simulink library "gmp_std_model_pck"  (R2024b)
settings: Solver=VariableStepAuto  StartTime=0.0  StopTime=10.0  RelTol=1e-3
undefined symbols (not defined in the file or in its folder): gcbh, sps_rtmsupport
libraries: spsSeriesRLCBranchLib x45, gmp_peripheral_utilities x32, spsVoltageMeasurementLib x21, spsSecondOrderFilterLib x19, spsMosfetLib x8, spsCurrentMeasurementLib x4, peripheral_utilities x3, gmp_fp_utilities x2, simulink x2
(part 3 of 5)

== system gmp_std_model_pck/Three Phase Bridge Ideal Current Measurement ==
  note: →
  note: Javnson
      | 2024.08.29
  note: GMP (General Motor Platform)
      | Simulink Toolkits
  note: current positive direction
  Trigger : Inport
  Ideal Current Measurement Module（ADC - Current）-U : gmp_peripheral_utilities/Ideal Current Measurement Module (ADC - Current)  ADC_GAIN=ADC_GAIN  ADC_BIT=ADC_BIT  ADC_REFERENCE=ADC_REFERENCE  ADC_BIAS=ADC_BIAS  ADC_INIT=ADC_INIT
      settings: SourceProductName=Virtual Peripheral Utilities
  Ideal Current Measurement Module（ADC - Current）-V : gmp_peripheral_utilities/Ideal Current Measurement Module (ADC - Current)  ADC_GAIN=ADC_GAIN  ADC_BIT=ADC_BIT  ADC_REFERENCE=ADC_REFERENCE  ADC_BIAS=ADC_BIAS  ADC_INIT=ADC_INIT
      settings: SourceProductName=Virtual Peripheral Utilities
  Ideal Current Measurement Module（ADC - Current）-W : gmp_peripheral_utilities/Ideal Current Measurement Module (ADC - Current)  ADC_GAIN=ADC_GAIN  ADC_BIT=ADC_BIT  ADC_REFERENCE=ADC_REFERENCE  ADC_BIAS=ADC_BIAS  ADC_INIT=ADC_INIT
      settings: SourceProductName=Virtual Peripheral Utilities
  Mux3 : Mux  Inputs=3
  Mux4 : Mux  Inputs=3
  Mux5 : Mux  Inputs=3
  A+ : PMIOPort  Side=Left
  B+ : PMIOPort  Port=2  Side=Left
  C+ : PMIOPort  Port=3  Side=Left
  a- : PMIOPort  Port=4  Side=Right
  b- : PMIOPort  Port=5  Side=Right
  c- : PMIOPort  Port=6  Side=Right
  Current ADC Sample Result : Outport
  Current ADC Scope(p.u.) : Outport  Port=2
  Current Real Value & HS : Outport  Port=3
  wires:
  [PhaseA_current] -> Mux3/1
  [PhaseB_current] -> Mux3/2
  [PhaseC_current] -> Mux3/3
  Mux3/1 -> Current ADC Sample Result/1
  [Ph_A_pu] -> Mux4/1
  [Ph_B_pu] -> Mux4/2
  [Ph_C_pu] -> Mux4/3
  Mux4/1 -> Current ADC Scope(p.u.)/1
  [Ph_B_HS] -> Mux5/2
  Mux5/1 -> Current Real Value & HS/1
  [Ph_C_HS] -> Mux5/3
  [Ph_A_HS] -> Mux5/1
  Trigger/1 -> Ideal Current Measurement Module（ADC - Current）-W/1, Ideal Current Measurement Module（ADC - Current）-V/1, Ideal Current Measurement Module（ADC - Current）-U/1
  Ideal Current Measurement Module（ADC - Current）-U/1 -> [PhaseA_current]
  Ideal Current Measurement Module（ADC - Current）-U/2 -> [Ph_A_pu]
  Ideal Current Measurement Module（ADC - Current）-U/3 -> [Ph_A_HS]
  Ideal Current Measurement Module（ADC - Current）-V/1 -> [PhaseB_current]
  Ideal Current Measurement Module（ADC - Current）-V/2 -> [Ph_B_pu]
  Ideal Current Measurement Module（ADC - Current）-V/3 -> [Ph_B_HS]
  Ideal Current Measurement Module（ADC - Current）-W/1 -> [PhaseC_current]
  Ideal Current Measurement Module（ADC - Current）-W/2 -> [Ph_C_pu]
  Ideal Current Measurement Module（ADC - Current）-W/3 -> [Ph_C_HS]
  connections:
  Ideal Current Measurement Module（ADC - Current）-U/LConn1 -- A+/RConn1
  Ideal Current Measurement Module（ADC - Current）-U/RConn1 -- a-/RConn1
  Ideal Current Measurement Module（ADC - Current）-V/RConn1 -- b-/RConn1
  Ideal Current Measurement Module（ADC - Current）-V/LConn1 -- B+/RConn1
  Ideal Current Measurement Module（ADC - Current）-W/RConn1 -- c-/RConn1
  Ideal Current Measurement Module（ADC - Current）-W/LConn1 -- C+/RConn1

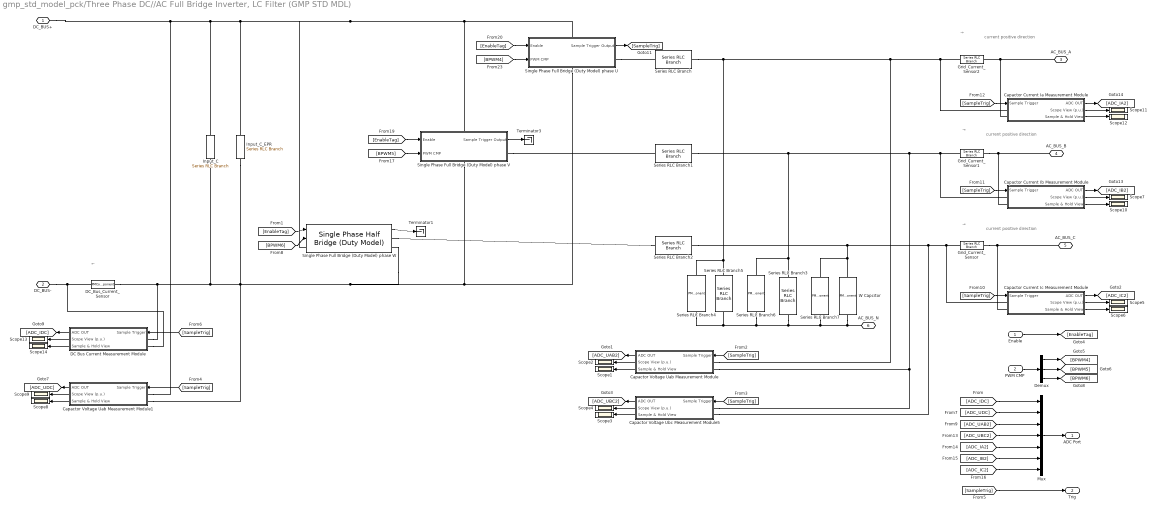
== system gmp_std_model_pck/Three Phase DC//AC Full Bridge Inverter, LC Filter (GMP STD MDL) ==
  note: current positive direction
  note: →
  note: current positive direction
  note: →
  note: current positive direction
  note: →
  note: ←
  Enable : Inport
  PWM CMP : Inport  Port=2
  Capactor Current Ia Measurement Module : Subsystem  AncestorBlock=peripheral_utilities/Ideal Voltage Measurement with filter Module(ADC - Voltage)  mask{ADC_GAIN=Grid_Current_Gain, ADC_BIT=ADC_Resolution, ADC_REFERENCE=GRID_CURRENT_ADC_REFERENCE, ADC_BIAS=GRID_CURRENT_ADC_BIAS, ADC_INIT=0, cut_frequency=GRID_CURRENT_ADC_CUT_FREQ}
      mask DialogControl DescGroupVar Prompt: Voltage Sample ADC Model
      mask DialogControl DescTextVar Prompt: This is a ideal Voltage Measurement Module.
      mask DialogControl Control2 Prompt: ADC(p.u.) = (real_voltage * ADC_GAIN + ADC_BIAS)/ADC_REFERENCE
      mask DialogControl Control11 Prompt: GMP CTL Simulink Utilities: virtual peripherals
      mask DialogControl ParameterGroupVar Prompt: Parameters:
      mask DialogControl Control4 Prompt: ADC Voltage Gain (Scale Factor):
      mask DialogControl Control5 Prompt: ADC resolution:
      mask DialogControl Control6 Prompt: ADC reference Voltage(V)
      mask DialogControl Control8 Prompt: ADC Bias Voltage(V)
      mask DialogControl Control7 Prompt: ADC Initial Voltage Output (V):
      mask DialogControl Control9 Prompt: Voltage Filter cut frequency (Hz):
      mask DialogControl Control10 Prompt: Generally, this value less than switch frequency / 10, greater than motor normal frequency * 3
  Capactor Current Ib Measurement Module : Subsystem  AncestorBlock=peripheral_utilities/Ideal Voltage Measurement with filter Module(ADC - Voltage)  mask{ADC_GAIN=Grid_Current_Gain, ADC_BIT=ADC_Resolution, ADC_REFERENCE=GRID_CURRENT_ADC_REFERENCE, ADC_BIAS=GRID_CURRENT_ADC_BIAS, ADC_INIT=0, cut_frequency=GRID_CURRENT_ADC_CUT_FREQ}
      mask DialogControl DescGroupVar Prompt: Voltage Sample ADC Model
      mask DialogControl DescTextVar Prompt: This is a ideal Voltage Measurement Module.
      mask DialogControl Control2 Prompt: ADC(p.u.) = (real_voltage * ADC_GAIN + ADC_BIAS)/ADC_REFERENCE
      mask DialogControl Control11 Prompt: GMP CTL Simulink Utilities: virtual peripherals
      mask DialogControl ParameterGroupVar Prompt: Parameters:
      mask DialogControl Control4 Prompt: ADC Voltage Gain (Scale Factor):
      mask DialogControl Control5 Prompt: ADC resolution:
      mask DialogControl Control6 Prompt: ADC reference Voltage(V)
      mask DialogControl Control8 Prompt: ADC Bias Voltage(V)
      mask DialogControl Control7 Prompt: ADC Initial Voltage Output (V):
      mask DialogControl Control9 Prompt: Voltage Filter cut frequency (Hz):
      mask DialogControl Control10 Prompt: Generally, this value less than switch frequency / 10, greater than motor normal frequency * 3
  Capactor Current Ic Measurement Module : Subsystem  AncestorBlock=peripheral_utilities/Ideal Voltage Measurement with filter Module(ADC - Voltage)  mask{ADC_GAIN=Grid_Current_Gain, ADC_BIT=ADC_Resolution, ADC_REFERENCE=GRID_CURRENT_ADC_REFERENCE, ADC_BIAS=GRID_CURRENT_ADC_BIAS, ADC_INIT=0, cut_frequency=GRID_CURRENT_ADC_CUT_FREQ}
      mask DialogControl DescGroupVar Prompt: Voltage Sample ADC Model
      mask DialogControl DescTextVar Prompt: This is a ideal Voltage Measurement Module.
      mask DialogControl Control2 Prompt: ADC(p.u.) = (real_voltage * ADC_GAIN + ADC_BIAS)/ADC_REFERENCE
      mask DialogControl Control11 Prompt: GMP CTL Simulink Utilities: virtual peripherals
      mask DialogControl ParameterGroupVar Prompt: Parameters:
      mask DialogControl Control4 Prompt: ADC Voltage Gain (Scale Factor):
      mask DialogControl Control5 Prompt: ADC resolution:
      mask DialogControl Control6 Prompt: ADC reference Voltage(V)
      mask DialogControl Control8 Prompt: ADC Bias Voltage(V)
      mask DialogControl Control7 Prompt: ADC Initial Voltage Output (V):
      mask DialogControl Control9 Prompt: Voltage Filter cut frequency (Hz):
      mask DialogControl Control10 Prompt: Generally, this value less than switch frequency / 10, greater than motor normal frequency * 3
  Capactor Voltage Uab Measurement Module : Subsystem  AncestorBlock=peripheral_utilities/Ideal Voltage Measurement with filter Module(ADC - Voltage)  mask{ADC_GAIN=AC_Voltage_Gain, ADC_BIT=ADC_Resolution, ADC_REFERENCE=AC_VOLTAGE_ADC_REFERENCE, ADC_BIAS=AC_VOLTAGE_ADC_BIAS, ADC_INIT=0, cut_frequency=AC_VOLTAGE_ADC_CUT_FREQ}
      mask DialogControl DescGroupVar Prompt: Voltage Sample ADC Model
      mask DialogControl DescTextVar Prompt: This is a ideal Voltage Measurement Module.
      mask DialogControl Control2 Prompt: ADC(p.u.) = (real_voltage * ADC_GAIN + ADC_BIAS)/ADC_REFERENCE
      mask DialogControl Control11 Prompt: GMP CTL Simulink Utilities: virtual peripherals
      mask DialogControl ParameterGroupVar Prompt: Parameters:
      mask DialogControl Control4 Prompt: ADC Voltage Gain (Scale Factor):
      mask DialogControl Control5 Prompt: ADC resolution:
      mask DialogControl Control6 Prompt: ADC reference Voltage(V)
      mask DialogControl Control8 Prompt: ADC Bias Voltage(V)
      mask DialogControl Control7 Prompt: ADC Initial Voltage Output (V):
      mask DialogControl Control9 Prompt: Voltage Filter cut frequency (Hz):
      mask DialogControl Control10 Prompt: Generally, this value less than switch frequency / 10, greater than motor normal frequency * 3
  Capactor Voltage Uab Measurement Module1 : Subsystem  mask{ADC_GAIN=DC_Voltage_Gain, ADC_BIT=ADC_Resolution, ADC_REFERENCE=DC_VOLTAGE_ADC_REFERENCE, ADC_BIAS=DC_VOLTAGE_ADC_BIAS, ADC_INIT=0, cut_frequency=DC_VOLTAGE_ADC_CUT_FREQ}
      mask DialogControl DescGroupVar Prompt: Voltage Sample ADC Model
      mask DialogControl DescTextVar Prompt: This is a ideal Voltage Measurement Module.
      mask DialogControl Control2 Prompt: ADC(p.u.) = (real_voltage * ADC_GAIN + ADC_BIAS)/ADC_REFERENCE
      mask DialogControl Control11 Prompt: GMP CTL Simulink Utilities: virtual peripherals
      mask DialogControl ParameterGroupVar Prompt: Parameters:
      mask DialogControl Control4 Prompt: ADC Voltage Gain (Scale Factor):
      mask DialogControl Control5 Prompt: ADC resolution:
      mask DialogControl Control6 Prompt: ADC reference Voltage(V)
      mask DialogControl Control8 Prompt: ADC Bias Voltage(V)
      mask DialogControl Control7 Prompt: ADC Initial Voltage Output (V):
      mask DialogControl Control9 Prompt: Voltage Filter cut frequency (Hz):
      mask DialogControl Control10 Prompt: Generally, this value less than switch frequency / 10, greater than motor normal frequency * 3
  Capactor Voltage Ubc Measurement Module5 : Subsystem  AncestorBlock=peripheral_utilities/Ideal Voltage Measurement with filter Module(ADC - Voltage)  mask{ADC_GAIN=AC_Voltage_Gain, ADC_BIT=ADC_Resolution, ADC_REFERENCE=AC_VOLTAGE_ADC_REFERENCE, ADC_BIAS=AC_VOLTAGE_ADC_BIAS, ADC_INIT=0, cut_frequency=AC_VOLTAGE_ADC_CUT_FREQ}
      mask DialogControl DescGroupVar Prompt: Voltage Sample ADC Model
      mask DialogControl DescTextVar Prompt: This is a ideal Voltage Measurement Module.
      mask DialogControl Control2 Prompt: ADC(p.u.) = (real_voltage * ADC_GAIN + ADC_BIAS)/ADC_REFERENCE
      mask DialogControl Control11 Prompt: GMP CTL Simulink Utilities: virtual peripherals
      mask DialogControl ParameterGroupVar Prompt: Parameters:
      mask DialogControl Control4 Prompt: ADC Voltage Gain (Scale Factor):
      mask DialogControl Control5 Prompt: ADC resolution:
      mask DialogControl Control6 Prompt: ADC reference Voltage(V)
      mask DialogControl Control8 Prompt: ADC Bias Voltage(V)
      mask DialogControl Control7 Prompt: ADC Initial Voltage Output (V):
      mask DialogControl Control9 Prompt: Voltage Filter cut frequency (Hz):
      mask DialogControl Control10 Prompt: Generally, this value less than switch frequency / 10, greater than motor normal frequency * 3
  DC Bus Current Measurement Module : Subsystem  mask{ADC_GAIN=DC_Current_Gain, ADC_BIT=ADC_Resolution, ADC_REFERENCE=DC_CURRENT_ADC_REFERENCE, ADC_BIAS=DC_CURRENT_ADC_BIAS, ADC_INIT=0, cut_frequency=DC_CURRENT_ADC_CUT_FREQ}
      mask DialogControl DescGroupVar Prompt: Voltage Sample ADC Model
      mask DialogControl DescTextVar Prompt: This is a ideal Voltage Measurement Module.
      mask DialogControl Control2 Prompt: ADC(p.u.) = (real_voltage * ADC_GAIN + ADC_BIAS)/ADC_REFERENCE
      mask DialogControl Control11 Prompt: GMP CTL Simulink Utilities: virtual peripherals
      mask DialogControl ParameterGroupVar Prompt: Parameters:
      mask DialogControl Control4 Prompt: ADC Voltage Gain (Scale Factor):
      mask DialogControl Control5 Prompt: ADC resolution:
      mask DialogControl Control6 Prompt: ADC reference Voltage(V)
      mask DialogControl Control8 Prompt: ADC Bias Voltage(V)
      mask DialogControl Control7 Prompt: ADC Initial Voltage Output (V):
      mask DialogControl Control9 Prompt: Voltage Filter cut frequency (Hz):
      mask DialogControl Control10 Prompt: Generally, this value less than switch frequency / 10, greater than motor normal frequency * 3
  DC_Bus_Current_Sensor : PMComponent  LoadFcn=sps_rtmsupport('LoadFcn',gcbh);  StartFcn=sps_rtmsupport('StartFcn',gcbh);  StopFcn=sps_rtmsupport('StopFcn',gcbh);  PhysicalDomain=powersysdomain  LeftPortType=p1  RightPortType=p1  LConnTagsString=__new0  RConnTagsString=__new0  mask(Series RLC Branch){BranchType=R, Resistance=DC_BUS_CURRENT_SENSOR_R, Inductance=1e-3, SetiL0=off, InitialCurrent=0, Capacitance=1e-6, Setx0=off, InitialVoltage=0, Measurements=None}
      mask prompts: BranchType "Branch type:"; Resistance "Resistance (Ohms):"; Inductance "Inductance (H):"; SetiL0 "Set the initial inductor current"; InitialCurrent "Inductor initial current (A):"; Capacitance "Capacitance (F):"; Setx0 "Set the initial capacitor voltage"; InitialVoltage "Capacitor initial voltage (V):"
      mask help:
      | Implements a series branch of RLC elements.
      | Use the 'Branch type' parameter to add or remove elements from the branch.
      mask init:
      | [s1,s2,s3,s4,r1,r2,l1,l2,c1,c2,c3,c4] = powericon('Series RLC Branch',Resistance,Inductance,Capacitance,BranchType);
      | powericon('RLCCback',gcb)
      | power_initmask();
      settings: CopyFcn=sps_rtmsupport('CopyFcn',gcbh);  DeleteFcn=sps_rtmsupport('DeleteFcn',gcbh);  UndoDeleteFcn=sps_rtmsupport('UndoDeleteFcn',gcbh);  ModelCloseFcn=sps_rtmsupport('ModelCloseFcn',gcbh);  PreSaveFcn=sps_rtmsupport('PreSaveFcn',gcbh);  PostSaveFcn=sps_rtmsupport('PostSaveFcn',gcbh);  NameChangeFcn=sps_rtmsupport('NameChangeFcn',gcbh);  PreCopyFcn=sps_rtmsupport('PreCopyFcn',gcbh);  OpenFcn=sps_rtmsupport('OpenFcn',gcbh, [1 4 7 9]);  CloseFcn=sps_rtmsupport('CloseFcn',gcbh);  PreDeleteFcn=sps_rtmsupport('PreDeleteFcn',gcbh);
      mask Help: helpview(psbhelp);
      mask TypeOptions BranchType: RLC | R | L | C | RL | RC | LC | Open circuit
      mask Callback BranchType: powericon('RLCCback',gcb)
      mask Callback Resistance: powericon('RLCCback',gcb)
      mask Callback Inductance: powericon('RLCCback',gcb)
      mask Callback SetiL0: powericon('RLCCback',gcb)
      mask Callback Capacitance: powericon('RLCCback',gcb)
      mask Callback Setx0: powericon('RLCCback',gcb)
      mask TypeOptions Measurements: None | Branch voltage | Branch current | Branch voltage and current
      mask Display:
      | plot(s1,s2,s3,s4,r1,r2*1.5,l1,l2*1.5,c1,c2*1.5,c3,c4*1.5)
      | color('red')
      | port_label('LConn',1,'+')
  Demux : Demux  Outputs=3
  Grid_Current_Sensor : spsSeriesRLCBranchLib/Series RLC Branch  LConnTagsString=__new0  RConnTagsString=__new0  BranchType=R  Resistance=GRID_CURRENT_SENSOR_R  Inductance=1e-3  SetiL0=off  InitialCurrent=0  Capacitance=1e-6  Setx0=off  InitialVoltage=0  Measurements=None
  Grid_Current_Sensor1 : spsSeriesRLCBranchLib/Series RLC Branch  LConnTagsString=__new0  RConnTagsString=__new0  BranchType=R  Resistance=GRID_CURRENT_SENSOR_R  Inductance=1e-3  SetiL0=off  InitialCurrent=0  Capacitance=1e-6  Setx0=off  InitialVoltage=0  Measurements=None
  Grid_Current_Sensor2 : spsSeriesRLCBranchLib/Series RLC Branch  LConnTagsString=__new0  RConnTagsString=__new0  BranchType=R  Resistance=GRID_CURRENT_SENSOR_R  Inductance=1e-3  SetiL0=off  InitialCurrent=0  Capacitance=1e-6  Setx0=off  InitialVoltage=0  Measurements=None
  Input_C : spsSeriesRLCBranchLib/Series RLC Branch  LConnTagsString=__new0  RConnTagsString=__new0  BranchType=RC  Resistance=DC_CAP_ESR  Inductance=1e-3  SetiL0=off  InitialCurrent=0  Capacitance=DC_CAP  Setx0=off  InitialVoltage=0  Measurements=None
  Input_C_EPR : spsSeriesRLCBranchLib/Series RLC Branch  LConnTagsString=__new0  RConnTagsString=__new0  BranchType=R  Resistance=DC_CAP_EPR  Inductance=1e-3  SetiL0=off  InitialCurrent=0  Capacitance=1e-6  Setx0=off  InitialVoltage=0  Measurements=None
  Mux : Mux  Inputs=7
  Scope{1..14} (14 alike) : Scope
  Series RLC Branch : spsSeriesRLCBranchLib/Series RLC Branch  LConnTagsString=__new0  RConnTagsString=__new0  BranchType=RL  Resistance=ACF_L_ESR  Inductance=ACF_L  SetiL0=off  InitialCurrent=0  Capacitance=1e-6  Setx0=off  InitialVoltage=0  Measurements=None
  Series RLC Branch1 : spsSeriesRLCBranchLib/Series RLC Branch  LConnTagsString=__new0  RConnTagsString=__new0  BranchType=RL  Resistance=ACF_L_ESR  Inductance=ACF_L  SetiL0=off  InitialCurrent=0  Capacitance=1e-6  Setx0=off  InitialVoltage=0  Measurements=None
  Series RLC Branch2 : spsSeriesRLCBranchLib/Series RLC Branch  LConnTagsString=__new0  RConnTagsString=__new0  BranchType=RL  Resistance=ACF_L_ESR  Inductance=ACF_L  SetiL0=off  InitialCurrent=0  Capacitance=1e-6  Setx0=off  InitialVoltage=0  Measurements=None
  Series RLC Branch3 : spsSeriesRLCBranchLib/Series RLC Branch  LConnTagsString=__new0  RConnTagsString=__new0  BranchType=RC  Resistance=ACF_C_ESR  Inductance=695e-6  SetiL0=off  InitialCurrent=0  Capacitance=ACF_C  Setx0=off  InitialVoltage=0  Measurements=None
  Series RLC Branch4 : PMComponent  LoadFcn=sps_rtmsupport('LoadFcn',gcbh);  StartFcn=sps_rtmsupport('StartFcn',gcbh);  StopFcn=sps_rtmsupport('StopFcn',gcbh);  PhysicalDomain=powersysdomain  LeftPortType=p1  RightPortType=p1  LConnTagsString=__new0  RConnTagsString=__new0  mask(Series RLC Branch){BranchType=R, Resistance=DC_CAP_EPR, Inductance=695e-6, SetiL0=off, InitialCurrent=0, Capacitance=ACF_C, Setx0=off, InitialVoltage=0, Measurements=None}
      mask prompts: BranchType "Branch type:"; Resistance "Resistance (Ohms):"; Inductance "Inductance (H):"; SetiL0 "Set the initial inductor current"; InitialCurrent "Inductor initial current (A):"; Capacitance "Capacitance (F):"; Setx0 "Set the initial capacitor voltage"; InitialVoltage "Capacitor initial voltage (V):"
      mask help:
      | Implements a series branch of RLC elements.
      | Use the 'Branch type' parameter to add or remove elements from the branch.
      mask init:
      | [s1,s2,s3,s4,r1,r2,l1,l2,c1,c2,c3,c4] = powericon('Series RLC Branch',Resistance,Inductance,Capacitance,BranchType);
      | powericon('RLCCback',gcb)
      | power_initmask();
      settings: CopyFcn=sps_rtmsupport('CopyFcn',gcbh);  DeleteFcn=sps_rtmsupport('DeleteFcn',gcbh);  UndoDeleteFcn=sps_rtmsupport('UndoDeleteFcn',gcbh);  ModelCloseFcn=sps_rtmsupport('ModelCloseFcn',gcbh);  PreSaveFcn=sps_rtmsupport('PreSaveFcn',gcbh);  PostSaveFcn=sps_rtmsupport('PostSaveFcn',gcbh);  NameChangeFcn=sps_rtmsupport('NameChangeFcn',gcbh);  PreCopyFcn=sps_rtmsupport('PreCopyFcn',gcbh);  OpenFcn=sps_rtmsupport('OpenFcn',gcbh, [1 4 7 9]);  CloseFcn=sps_rtmsupport('CloseFcn',gcbh);  PreDeleteFcn=sps_rtmsupport('PreDeleteFcn',gcbh);
      mask Help: helpview(psbhelp);
      mask TypeOptions BranchType: RLC | R | L | C | RL | RC | LC | Open circuit
      mask Callback BranchType: powericon('RLCCback',gcb)
      mask Callback Resistance: powericon('RLCCback',gcb)
      mask Callback Inductance: powericon('RLCCback',gcb)
      mask Callback SetiL0: powericon('RLCCback',gcb)
      mask Callback Capacitance: powericon('RLCCback',gcb)
      mask Callback Setx0: powericon('RLCCback',gcb)
      mask TypeOptions Measurements: None | Branch voltage | Branch current | Branch voltage and current
      mask Display:
      | plot(s1,s2,s3,s4,r1,r2*1.5,l1,l2*1.5,c1,c2*1.5,c3,c4*1.5)
      | color('red')
      | port_label('LConn',1,'+')
  Series RLC Branch5 : spsSeriesRLCBranchLib/Series RLC Branch  LConnTagsString=__new0  RConnTagsString=__new0  BranchType=RC  Resistance=ACF_C_ESR  Inductance=695e-6  SetiL0=off  InitialCurrent=0  Capacitance=ACF_C  Setx0=off  InitialVoltage=0  Measurements=None
  Series RLC Branch6 : PMComponent  LoadFcn=sps_rtmsupport('LoadFcn',gcbh);  StartFcn=sps_rtmsupport('StartFcn',gcbh);  StopFcn=sps_rtmsupport('StopFcn',gcbh);  PhysicalDomain=powersysdomain  LeftPortType=p1  RightPortType=p1  LConnTagsString=__new0  RConnTagsString=__new0  mask(Series RLC Branch){BranchType=R, Resistance=DC_CAP_EPR, Inductance=695e-6, SetiL0=off, InitialCurrent=0, Capacitance=ACF_C, Setx0=off, InitialVoltage=0, Measurements=None}
      mask prompts: BranchType "Branch type:"; Resistance "Resistance (Ohms):"; Inductance "Inductance (H):"; SetiL0 "Set the initial inductor current"; InitialCurrent "Inductor initial current (A):"; Capacitance "Capacitance (F):"; Setx0 "Set the initial capacitor voltage"; InitialVoltage "Capacitor initial voltage (V):"
      mask help:
      | Implements a series branch of RLC elements.
      | Use the 'Branch type' parameter to add or remove elements from the branch.
      mask init:
      | [s1,s2,s3,s4,r1,r2,l1,l2,c1,c2,c3,c4] = powericon('Series RLC Branch',Resistance,Inductance,Capacitance,BranchType);
      | powericon('RLCCback',gcb)
      | power_initmask();
      settings: CopyFcn=sps_rtmsupport('CopyFcn',gcbh);  DeleteFcn=sps_rtmsupport('DeleteFcn',gcbh);  UndoDeleteFcn=sps_rtmsupport('UndoDeleteFcn',gcbh);  ModelCloseFcn=sps_rtmsupport('ModelCloseFcn',gcbh);  PreSaveFcn=sps_rtmsupport('PreSaveFcn',gcbh);  PostSaveFcn=sps_rtmsupport('PostSaveFcn',gcbh);  NameChangeFcn=sps_rtmsupport('NameChangeFcn',gcbh);  PreCopyFcn=sps_rtmsupport('PreCopyFcn',gcbh);  OpenFcn=sps_rtmsupport('OpenFcn',gcbh, [1 4 7 9]);  CloseFcn=sps_rtmsupport('CloseFcn',gcbh);  PreDeleteFcn=sps_rtmsupport('PreDeleteFcn',gcbh);
      mask Help: helpview(psbhelp);
      mask TypeOptions BranchType: RLC | R | L | C | RL | RC | LC | Open circuit
      mask Callback BranchType: powericon('RLCCback',gcb)
      mask Callback Resistance: powericon('RLCCback',gcb)
      mask Callback Inductance: powericon('RLCCback',gcb)
      mask Callback SetiL0: powericon('RLCCback',gcb)
      mask Callback Capacitance: powericon('RLCCback',gcb)
      mask Callback Setx0: powericon('RLCCback',gcb)
      mask TypeOptions Measurements: None | Branch voltage | Branch current | Branch voltage and current
      mask Display:
      | plot(s1,s2,s3,s4,r1,r2*1.5,l1,l2*1.5,c1,c2*1.5,c3,c4*1.5)
      | color('red')
      | port_label('LConn',1,'+')
  Series RLC Branch7 : PMComponent  LoadFcn=sps_rtmsupport('LoadFcn',gcbh);  StartFcn=sps_rtmsupport('StartFcn',gcbh);  StopFcn=sps_rtmsupport('StopFcn',gcbh);  PhysicalDomain=powersysdomain  LeftPortType=p1  RightPortType=p1  LConnTagsString=__new0  RConnTagsString=__new0  mask(Series RLC Branch){BranchType=R, Resistance=DC_CAP_EPR, Inductance=695e-6, SetiL0=off, InitialCurrent=0, Capacitance=ACF_C, Setx0=off, InitialVoltage=0, Measurements=None}
      mask prompts: BranchType "Branch type:"; Resistance "Resistance (Ohms):"; Inductance "Inductance (H):"; SetiL0 "Set the initial inductor current"; InitialCurrent "Inductor initial current (A):"; Capacitance "Capacitance (F):"; Setx0 "Set the initial capacitor voltage"; InitialVoltage "Capacitor initial voltage (V):"
      mask help:
      | Implements a series branch of RLC elements.
      | Use the 'Branch type' parameter to add or remove elements from the branch.
      mask init:
      | [s1,s2,s3,s4,r1,r2,l1,l2,c1,c2,c3,c4] = powericon('Series RLC Branch',Resistance,Inductance,Capacitance,BranchType);
      | powericon('RLCCback',gcb)
      | power_initmask();
      settings: CopyFcn=sps_rtmsupport('CopyFcn',gcbh);  DeleteFcn=sps_rtmsupport('DeleteFcn',gcbh);  UndoDeleteFcn=sps_rtmsupport('UndoDeleteFcn',gcbh);  ModelCloseFcn=sps_rtmsupport('ModelCloseFcn',gcbh);  PreSaveFcn=sps_rtmsupport('PreSaveFcn',gcbh);  PostSaveFcn=sps_rtmsupport('PostSaveFcn',gcbh);  NameChangeFcn=sps_rtmsupport('NameChangeFcn',gcbh);  PreCopyFcn=sps_rtmsupport('PreCopyFcn',gcbh);  OpenFcn=sps_rtmsupport('OpenFcn',gcbh, [1 4 7 9]);  CloseFcn=sps_rtmsupport('CloseFcn',gcbh);  PreDeleteFcn=sps_rtmsupport('PreDeleteFcn',gcbh);
      mask Help: helpview(psbhelp);
      mask TypeOptions BranchType: RLC | R | L | C | RL | RC | LC | Open circuit
      mask Callback BranchType: powericon('RLCCback',gcb)
      mask Callback Resistance: powericon('RLCCback',gcb)
      mask Callback Inductance: powericon('RLCCback',gcb)
      mask Callback SetiL0: powericon('RLCCback',gcb)
      mask Callback Capacitance: powericon('RLCCback',gcb)
      mask Callback Setx0: powericon('RLCCback',gcb)
      mask TypeOptions Measurements: None | Branch voltage | Branch current | Branch voltage and current
      mask Display:
      | plot(s1,s2,s3,s4,r1,r2*1.5,l1,l2*1.5,c1,c2*1.5,c3,c4*1.5)
      | color('red')
      | port_label('LConn',1,'+')
  Single Phase Full Bridge (Duty Model) phase U : Subsystem  mask{fswitch=fswitch, CMP_MAX=CMP_MAX, Deadband_Upper=Deadband_Upper, Deadband_Lower=Deadband_Lower, Deadband_us=NaN, phase_shift=0, R_mosfet_on=0.1, Lon=0, Rd=0.01, Vf=0.3, Rs=1e5, Cs=inf}
      mask init:
      | calculate_deadband(gcb, 'Deadband_Upper', 'Deadband_Lower',	'CMP_MAX', 'fswitch', 'Deadband_us');
      settings: PortSchema="{\"entries\":[{\"content\":{\"sides\":[{\"content\":{\"connectorIds\":[\"In1\",\"In2\"]},\"type\":\"ConnectorPlacement.EquallySpacedRectSide\",\"uuid\":\"20beeabc-b0ca-4337-b227-c7f02abd15d8\"},{\"content\":{\"connectorIds\":[\"Out1\",\"RConn1\"],\"side\":\"RIGHT\"},\"type\":\"ConnectorPlacement.EquallySpacedRectSide\",\"uuid\":\"a7923383-ac55-4621-ad1d-4d067c1fb84d\"},{\"content\":{\"connectorIds\":[\"LConn1\"],\"side\":\"TOP\"},\"type\":\"ConnectorPlacement.EquallySpacedRectSide\",\"uuid\":\"661bf0ae-1c96-4de8-96aa-28c06a0a56db\"},{\"content\":{\"connectorIds\":[\"RConn2\"],\"side\":\"BOTTOM\"},\"type\":\"ConnectorPlacement.EquallySpacedRectSide\",\"uuid\":\"fc2f6321-5787-4e1a-b5a2-65ed34db36b5\"}]},\"type\":\"ConnectorPlacement.EquallySpacedConnector\",\"uuid\":\"e2219b16-0a50-43ef-8183-c55a35d5a2a0\"}],\"packageUris\":[\"http://schema.mathworks.com/mf0/Connector/R2020b\"],\"version\":\"1.0\"}"
      mask Callback fswitch: calculate_deadband(gcb, 'Deadband_Upper', 'Deadband_Lower',	'CMP_MAX', 'fswitch', 'Deadband_us');
      mask Callback CMP_MAX: calculate_deadband(gcb, 'Deadband_Upper', 'Deadband_Lower',	'CMP_MAX', 'fswitch', 'Deadband_us');
      mask Callback Deadband_Upper: calculate_deadband(gcb, 'Deadband_Upper', 'Deadband_Lower',	'CMP_MAX', 'fswitch', 'Deadband_us');
      mask Callback Deadband_Lower: calculate_deadband(gcb, 'Deadband_Upper', 'Deadband_Lower',	'CMP_MAX', 'fswitch', 'Deadband_us');
      mask DialogControl DescGroupVar Prompt: Half Bridge With PWM Module
      mask DialogControl Control14 Prompt: GMP CTL Simulink Utilities: virtual peripherals
      mask DialogControl DescTextVar Prompt: This module provide a PWM (with deadband), and a MOSFET half bridge.
      mask DialogControl Container5 Prompt: PWM Modulator
      mask DialogControl ParameterGroupVar Prompt: PWM module parameters
      mask DialogControl Control2 Prompt: PWM Frequency (Hz):
      mask DialogControl Control3 Prompt: Full Scale PWM Compare value:
      mask DialogControl Control4 Prompt: (whole period is 2 * CMP_MAX ticks)
      mask DialogControl Control5 Prompt: Deadband Range Set (CMP Value):
      mask DialogControl Control6 Prompt: Single side deadband time: DEADBAND_CMP/2/CMP_MAX/fswitch
      mask DialogControl Control15 Prompt: Calculated Deadband, us
      mask DialogControl Control13 Prompt: Initial Phase Shift, unit rad
      mask DialogControl Container6 Prompt: MOSFET
      mask DialogControl Container3 Prompt: MOSFET parameters
      mask DialogControl Control7 Prompt: Rds(on), unit Ohm
      mask DialogControl Control8 Prompt: Internal diode inducctance, unit H
      mask DialogControl Control9 Prompt: Internal diode resistance Rd, unit Ohm
      mask DialogControl Control10 Prompt: Internal diode forward voltage Vf, unit V
      mask DialogControl Control11 Prompt: Snubber resistance Rs, unit ohm
      mask DialogControl Control12 Prompt: Snubber Capacitance Cs, unit F
  Single Phase Full Bridge (Duty Model) phase V : Subsystem  mask{fswitch=fswitch, CMP_MAX=CMP_MAX, Deadband_Upper=Deadband_Upper, Deadband_Lower=Deadband_Lower, Deadband_us=NaN, phase_shift=0, R_mosfet_on=0.1, Lon=0, Rd=0.01, Vf=0.3, Rs=1e5, Cs=inf}
      mask init:
      | calculate_deadband(gcb, 'Deadband_Upper', 'Deadband_Lower',	'CMP_MAX', 'fswitch', 'Deadband_us');
      settings: PortSchema="{\"entries\":[{\"content\":{\"sides\":[{\"content\":{\"connectorIds\":[\"In1\",\"In2\"]},\"type\":\"ConnectorPlacement.EquallySpacedRectSide\",\"uuid\":\"20beeabc-b0ca-4337-b227-c7f02abd15d8\"},{\"content\":{\"connectorIds\":[\"Out1\",\"RConn1\"],\"side\":\"RIGHT\"},\"type\":\"ConnectorPlacement.EquallySpacedRectSide\",\"uuid\":\"a7923383-ac55-4621-ad1d-4d067c1fb84d\"},{\"content\":{\"connectorIds\":[\"LConn1\"],\"side\":\"TOP\"},\"type\":\"ConnectorPlacement.EquallySpacedRectSide\",\"uuid\":\"661bf0ae-1c96-4de8-96aa-28c06a0a56db\"},{\"content\":{\"connectorIds\":[\"RConn2\"],\"side\":\"BOTTOM\"},\"type\":\"ConnectorPlacement.EquallySpacedRectSide\",\"uuid\":\"fc2f6321-5787-4e1a-b5a2-65ed34db36b5\"}]},\"type\":\"ConnectorPlacement.EquallySpacedConnector\",\"uuid\":\"e2219b16-0a50-43ef-8183-c55a35d5a2a0\"}],\"packageUris\":[\"http://schema.mathworks.com/mf0/Connector/R2020b\"],\"version\":\"1.0\"}"
      mask Callback fswitch: calculate_deadband(gcb, 'Deadband_Upper', 'Deadband_Lower',	'CMP_MAX', 'fswitch', 'Deadband_us');
      mask Callback CMP_MAX: calculate_deadband(gcb, 'Deadband_Upper', 'Deadband_Lower',	'CMP_MAX', 'fswitch', 'Deadband_us');
      mask Callback Deadband_Upper: calculate_deadband(gcb, 'Deadband_Upper', 'Deadband_Lower',	'CMP_MAX', 'fswitch', 'Deadband_us');
      mask Callback Deadband_Lower: calculate_deadband(gcb, 'Deadband_Upper', 'Deadband_Lower',	'CMP_MAX', 'fswitch', 'Deadband_us');
      mask DialogControl DescGroupVar Prompt: Half Bridge With PWM Module
      mask DialogControl Control14 Prompt: GMP CTL Simulink Utilities: virtual peripherals
      mask DialogControl DescTextVar Prompt: This module provide a PWM (with deadband), and a MOSFET half bridge.
      mask DialogControl Container5 Prompt: PWM Modulator
      mask DialogControl ParameterGroupVar Prompt: PWM module parameters
      mask DialogControl Control2 Prompt: PWM Frequency (Hz):
      mask DialogControl Control3 Prompt: Full Scale PWM Compare value:
      mask DialogControl Control4 Prompt: (whole period is 2 * CMP_MAX ticks)
      mask DialogControl Control5 Prompt: Deadband Range Set (CMP Value):
      mask DialogControl Control6 Prompt: Single side deadband time: DEADBAND_CMP/2/CMP_MAX/fswitch
      mask DialogControl Control15 Prompt: Calculated Deadband, us
      mask DialogControl Control13 Prompt: Initial Phase Shift, unit rad
      mask DialogControl Container6 Prompt: MOSFET
      mask DialogControl Container3 Prompt: MOSFET parameters
      mask DialogControl Control7 Prompt: Rds(on), unit Ohm
      mask DialogControl Control8 Prompt: Internal diode inducctance, unit H
      mask DialogControl Control9 Prompt: Internal diode resistance Rd, unit Ohm
      mask DialogControl Control10 Prompt: Internal diode forward voltage Vf, unit V
      mask DialogControl Control11 Prompt: Snubber resistance Rs, unit ohm
      mask DialogControl Control12 Prompt: Snubber Capacitance Cs, unit F
  Single Phase Full Bridge (Duty Model) phase W : gmp_peripheral_utilities/Single Phase Half Bridge (Duty Model)  fswitch=fswitch  CMP_MAX=CMP_MAX  Deadband_Upper=Deadband_Upper  Deadband_Lower=Deadband_Lower  Deadband_us=NaN  phase_shift=0  R_mosfet_on=0.1  Lon=0  Rd=0.01  Vf=0.3  Rs=1e5  Cs=inf
      settings: SourceProductName=Virtual Peripheral Utilities
  Terminator1 : Terminator
  Terminator3 : Terminator
  W Capcitor : PMComponent  LoadFcn=sps_rtmsupport('LoadFcn',gcbh);  StartFcn=sps_rtmsupport('StartFcn',gcbh);  StopFcn=sps_rtmsupport('StopFcn',gcbh);  PhysicalDomain=powersysdomain  LeftPortType=p1  RightPortType=p1  LConnTagsString=__new0  RConnTagsString=__new0  mask(Series RLC Branch){BranchType=RC, Resistance=ACF_C_ESR, Inductance=695e-6, SetiL0=off, InitialCurrent=0, Capacitance=ACF_C, Setx0=off, InitialVoltage=0, Measurements=None}
      mask prompts: BranchType "Branch type:"; Resistance "Resistance (Ohms):"; Inductance "Inductance (H):"; SetiL0 "Set the initial inductor current"; InitialCurrent "Inductor initial current (A):"; Capacitance "Capacitance (F):"; Setx0 "Set the initial capacitor voltage"; InitialVoltage "Capacitor initial voltage (V):"
      mask help:
      | Implements a series branch of RLC elements.
      | Use the 'Branch type' parameter to add or remove elements from the branch.
      mask init:
      | [s1,s2,s3,s4,r1,r2,l1,l2,c1,c2,c3,c4] = powericon('Series RLC Branch',Resistance,Inductance,Capacitance,BranchType);
      | powericon('RLCCback',gcb)
      | power_initmask();
      settings: CopyFcn=sps_rtmsupport('CopyFcn',gcbh);  DeleteFcn=sps_rtmsupport('DeleteFcn',gcbh);  UndoDeleteFcn=sps_rtmsupport('UndoDeleteFcn',gcbh);  ModelCloseFcn=sps_rtmsupport('ModelCloseFcn',gcbh);  PreSaveFcn=sps_rtmsupport('PreSaveFcn',gcbh);  PostSaveFcn=sps_rtmsupport('PostSaveFcn',gcbh);  NameChangeFcn=sps_rtmsupport('NameChangeFcn',gcbh);  PreCopyFcn=sps_rtmsupport('PreCopyFcn',gcbh);  OpenFcn=sps_rtmsupport('OpenFcn',gcbh, [1 4 7 9]);  CloseFcn=sps_rtmsupport('CloseFcn',gcbh);  PreDeleteFcn=sps_rtmsupport('PreDeleteFcn',gcbh);
      mask Help: helpview(psbhelp);
      mask TypeOptions BranchType: RLC | R | L | C | RL | RC | LC | Open circuit
      mask Callback BranchType: powericon('RLCCback',gcb)
      mask Callback Resistance: powericon('RLCCback',gcb)
      mask Callback Inductance: powericon('RLCCback',gcb)
      mask Callback SetiL0: powericon('RLCCback',gcb)
      mask Callback Capacitance: powericon('RLCCback',gcb)
      mask Callback Setx0: powericon('RLCCback',gcb)
      mask TypeOptions Measurements: None | Branch voltage | Branch current | Branch voltage and current
      mask Display:
      | plot(s1,s2,s3,s4,r1,r2*1.5,l1,l2*1.5,c1,c2*1.5,c3,c4*1.5)
      | color('red')
      | port_label('LConn',1,'+')
  DC_BUS+ : PMIOPort  Side=Left
  DC_BUS- : PMIOPort  Port=2  Side=Left
  AC_BUS_A : PMIOPort  Port=3  Side=Right
  AC_BUS_B : PMIOPort  Port=4  Side=Right
  AC_BUS_C : PMIOPort  Port=5  Side=Right
  AC_BUS_N : PMIOPort  Port=6  Side=Right
  ADC Port : Outport
  Trig : Outport  Port=2
  wires:
  Single Phase Full Bridge (Duty Model) phase U/1(Sample Trigger Output) -> [SampleTrig]
  [BPWM4] -> Single Phase Full Bridge (Duty Model) phase U/2(PWM CMP)
  [EnableTag] -> Single Phase Full Bridge (Duty Model) phase U/1(Enable)
  Single Phase Full Bridge (Duty Model) phase V/1(Sample Trigger Output) -> Terminator3/1
  [EnableTag] -> Single Phase Full Bridge (Duty Model) phase V/1(Enable)
  [BPWM5] -> Single Phase Full Bridge (Duty Model) phase V/2(PWM CMP)
  Enable/1 -> [EnableTag]
  PWM CMP/1 -> Demux/1
  Demux/1 -> [BPWM4]
  Demux/2 -> [BPWM5]
  Mux/1 -> ADC Port/1
  [SampleTrig] -> Trig/1
  [BPWM6] -> Single Phase Full Bridge (Duty Model) phase W/2
  Demux/3 -> [BPWM6]
  Capactor Current Ic Measurement Module/1(ADC OUT) -> [ADC_IC2]
  Capactor Current Ic Measurement Module/2(Scope View (p.u.)) -> Scope5/1
  Capactor Current Ic Measurement Module/3(Sample & Hold View) -> Scope6/1
  [SampleTrig] -> Capactor Current Ic Measurement Module/1(Sample Trigger)
  Capactor Current Ib Measurement Module/2(Scope View (p.u.)) -> Scope7/1
  [SampleTrig] -> Capactor Current Ib Measurement Module/1(Sample Trigger)
  Capactor Current Ib Measurement Module/3(Sample & Hold View) -> Scope10/1
  Capactor Current Ib Measurement Module/1(ADC OUT) -> [ADC_IB2]
  Capactor Current Ia Measurement Module/2(Scope View (p.u.)) -> Scope11/1
  [SampleTrig] -> Capactor Current Ia Measurement Module/1(Sample Trigger)
  Capactor Current Ia Measurement Module/3(Sample & Hold View) -> Scope12/1
  Capactor Current Ia Measurement Module/1(ADC OUT) -> [ADC_IA2]
  Single Phase Full Bridge (Duty Model) phase W/1 -> Terminator1/1
  [EnableTag] -> Single Phase Full Bridge (Duty Model) phase W/1
  [SampleTrig] -> Capactor Voltage Uab Measurement Module/1(Sample Trigger)
  Capactor Voltage Uab Measurement Module/2(Scope View (p.u.)) -> Scope2/1
  Capactor Voltage Uab Measurement Module/3(Sample & Hold View) -> Scope1/1
  Capactor Voltage Uab Measurement Module/1(ADC OUT) -> [ADC_UAB2]
  Capactor Voltage Ubc Measurement Module5/1(ADC OUT) -> [ADC_UBC2]
  Capactor Voltage Ubc Measurement Module5/3(Sample & Hold View) -> Scope3/1
  [SampleTrig] -> Capactor Voltage Ubc Measurement Module5/1(Sample Trigger)
  Capactor Voltage Ubc Measurement Module5/2(Scope View (p.u.)) -> Scope4/1
  [SampleTrig] -> Capactor Voltage Uab Measurement Module1/1(Sample Trigger)
  Capactor Voltage Uab Measurement Module1/1(ADC OUT) -> [ADC_UDC]
  Capactor Voltage Uab Measurement Module1/2(Scope View (p.u.)) -> Scope9/1
  Capactor Voltage Uab Measurement Module1/3(Sample & Hold View) -> Scope8/1
  [SampleTrig] -> DC Bus Current Measurement Module/1(Sample Trigger)
  DC Bus Current Measurement Module/3(Sample & Hold View) -> Scope14/1
  DC Bus Current Measurement Module/2(Scope View (p.u.)) -> Scope13/1
  DC Bus Current Measurement Module/1(ADC OUT) -> [ADC_IDC]
  [ADC_IDC] -> Mux/1
  [ADC_UDC] -> Mux/2
  [ADC_UAB2] -> Mux/3
  [ADC_UBC2] -> Mux/4
  [ADC_IA2] -> Mux/5
  [ADC_IB2] -> Mux/6
  [ADC_IC2] -> Mux/7
  connections:
  Input_C/RConn1 -- Capactor Voltage Uab Measurement Module1/LConn2 -- Input_C_EPR/RConn1 -- Single Phase Full Bridge (Duty Model) phase W/RConn2 -- Single Phase Full Bridge (Duty Model) phase U/RConn2 -- Single Phase Full Bridge (Duty Model) phase V/RConn2 -- DC Bus Current Measurement Module/LConn1 -- DC_Bus_Current_Sensor/LConn1
  DC_BUS+/RConn1 -- Input_C/LConn1 -- Input_C_EPR/LConn1 -- Single Phase Full Bridge (Duty Model) phase W/LConn1 -- Single Phase Full Bridge (Duty Model) phase U/LConn1 -- Single Phase Full Bridge (Duty Model) phase V/LConn1 -- Capactor Voltage Uab Measurement Module1/LConn1
  Grid_Current_Sensor1/RConn1 -- Series RLC Branch6/RConn1 -- Series RLC Branch3/RConn1 -- Series RLC Branch1/RConn1 -- Capactor Voltage Ubc Measurement Module5/LConn1 -- Capactor Voltage Uab Measurement Module/LConn2 -- Capactor Current Ib Measurement Module/LConn1
  Capactor Current Ic Measurement Module/LConn1 -- Grid_Current_Sensor/RConn1 -- Capactor Voltage Ubc Measurement Module5/LConn2 -- Series RLC Branch7/RConn1 -- W Capcitor/RConn1 -- Series RLC Branch2/RConn1
  Grid_Current_Sensor/LConn1 -- AC_BUS_C/RConn1 -- Capactor Current Ic Measurement Module/LConn2
  Grid_Current_Sensor1/LConn1 -- Capactor Current Ib Measurement Module/LConn2 -- AC_BUS_B/RConn1
  AC_BUS_A/RConn1 -- Capactor Current Ia Measurement Module/LConn2 -- Grid_Current_Sensor2/LConn1
  AC_BUS_N/RConn1 -- Series RLC Branch7/LConn1 -- Series RLC Branch3/LConn1 -- Series RLC Branch6/LConn1 -- Series RLC Branch4/LConn1 -- Series RLC Branch5/LConn1 -- W Capcitor/LConn1
  Single Phase Full Bridge (Duty Model) phase U/RConn1 -- Series RLC Branch/LConn1
  Grid_Current_Sensor2/RConn1 -- Capactor Voltage Uab Measurement Module/LConn1 -- Series RLC Branch/RConn1 -- Series RLC Branch4/RConn1 -- Series RLC Branch5/RConn1 -- Capactor Current Ia Measurement Module/LConn1
  Single Phase Full Bridge (Duty Model) phase W/RConn1 -- Series RLC Branch2/LConn1
  Single Phase Full Bridge (Duty Model) phase V/RConn1 -- Series RLC Branch1/LConn1
  DC_BUS-/RConn1 -- DC Bus Current Measurement Module/LConn2 -- DC_Bus_Current_Sensor/RConn1

== system gmp_std_model_pck/Three Phase Driver Model ==
  note: Javnson
      | 2024.08.29
  note: GMP (General Motor Platform)
      | Simulink Toolkits
  Enable : Inport
  PWM U : Inport  Port=2
  PWM V : Inport  Port=3
  PWM W : Inport  Port=4
  Single Phase Half Bridge U : gmp_peripheral_utilities/Single Phase Half Bridge (Duty Model)  fswitch=fswitch  CMP_MAX=CMP_MAX  Deadband_Upper=Deadband_Upper  Deadband_Lower=Deadband_Lower  Deadband_us=NaN  phase_shift=0  R_mosfet_on=R_mosfet_on  Lon=Lon  Rd=Rd  Vf=Vf  Rs=Rs  Cs=Cs
      settings: SourceProductName=Virtual Peripheral Utilities
  Single Phase Half Bridge V : gmp_peripheral_utilities/Single Phase Half Bridge (Duty Model)  fswitch=fswitch  CMP_MAX=CMP_MAX  Deadband_Upper=Deadband_Upper  Deadband_Lower=Deadband_Lower  Deadband_us=NaN  phase_shift=0  R_mosfet_on=R_mosfet_on  Lon=Lon  Rd=Rd  Vf=Vf  Rs=Rs  Cs=Cs
      settings: SourceProductName=Virtual Peripheral Utilities
  Single Phase Half Bridge W : gmp_peripheral_utilities/Single Phase Half Bridge (Duty Model)  fswitch=fswitch  CMP_MAX=CMP_MAX  Deadband_Upper=Deadband_Upper  Deadband_Lower=Deadband_Lower  Deadband_us=NaN  phase_shift=0  R_mosfet_on=R_mosfet_on  Lon=Lon  Rd=Rd  Vf=Vf  Rs=Rs  Cs=Cs
      settings: SourceProductName=Virtual Peripheral Utilities
  Terminator : Terminator
  Terminator1 : Terminator
  U : PMIOPort  Side=Right
  V : PMIOPort  Port=2  Side=Right
  W : PMIOPort  Port=3  Side=Right
  Pwr+ : PMIOPort  Port=4  Side=Right
  Pwr- : PMIOPort  Port=5  Side=Right
  Sample Trigger Output : Outport
  wires:
  PWM W/1 -> Single Phase Half Bridge W/2
  Single Phase Half Bridge W/1 -> Terminator1/1
  Enable/1 -> Single Phase Half Bridge U/1, Single Phase Half Bridge W/1, Single Phase Half Bridge V/1
  Single Phase Half Bridge V/1 -> Terminator/1
  Single Phase Half Bridge U/1 -> Sample Trigger Output/1
  PWM U/1 -> Single Phase Half Bridge U/2
  PWM V/1 -> Single Phase Half Bridge V/2
  connections:
  Single Phase Half Bridge V/LConn1 -- Single Phase Half Bridge U/LConn1 -- Pwr+/RConn1 -- Single Phase Half Bridge W/LConn1
  Single Phase Half Bridge V/RConn2 -- Single Phase Half Bridge U/RConn2 -- Pwr-/RConn1 -- Single Phase Half Bridge W/RConn2
  Single Phase Half Bridge V/RConn1 -- V/RConn1
  Single Phase Half Bridge W/RConn1 -- W/RConn1
  Single Phase Half Bridge U/RConn1 -- U/RConn1
